simulink subsystem "RT_HubLinearAndAngularVelocity"  (R2025a)
settings: Solver=VariableStepAuto  StartTime=0.0  StopTime=10.0  RelTol=1e-3
settings Model: DataDictionary=Helicopter.sldd  EnableAccessToBaseWorkspace=off  DefaultTestHarness=RT_HubLinearAndAngularVelocity_Harness6  Creator=Admin  LastModifiedBy=Admin

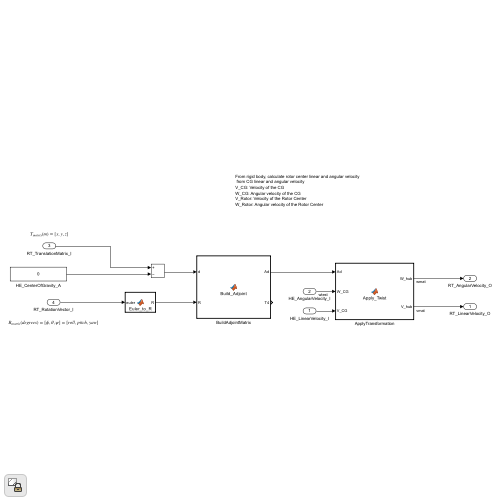
[thumbnail: Simulink's stored preview of the top-level diagram]
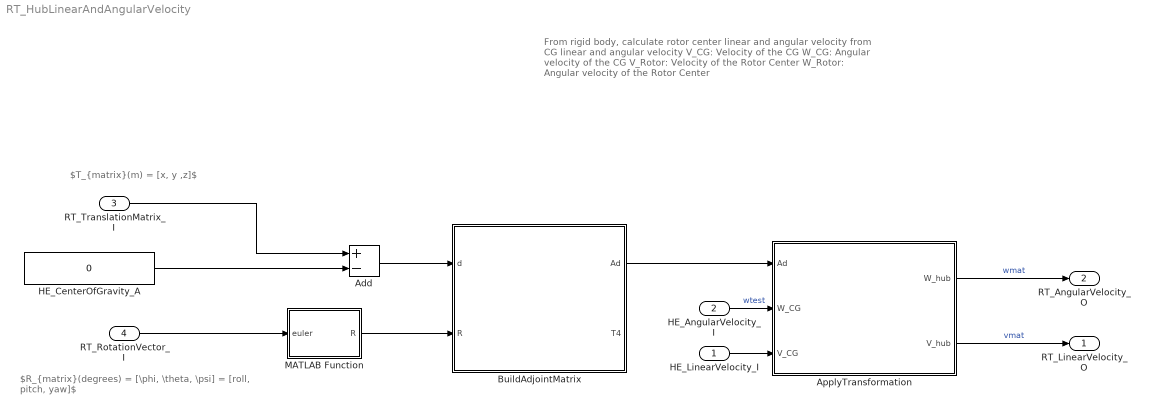
== system RT_HubLinearAndAngularVelocity ==
  note: From rigid body, calculate rotor center linear and angular velocity
      |  from CG linear and angular velocity
      | V_CG: Velocity of the CG
      | W_CG: Angular velocity of the CG
      | V_Rotor: Velocity of the Rotor Center
      | W_Rotor: Angular velocity of the Rotor Center
  note: $R_{matrix}(degrees) = [\phi, \theta, \psi] = [roll, pitch, yaw]$
  note: $T_{matrix}(m) = [x, y ,z]$
  HE_LinearVelocity_I : Inport
  HE_AngularVelocity_I : Inport  Port=2
  RT_TranslationMatrix_I : Inport  Port=3
  RT_RotationVector_I : Inport  Port=4
  Add : Sum  Inputs=+-
  ApplyTransformation : MATLAB Function  TreatAsAtomicUnit=on
  BuildAdjointMatrix : MATLAB Function  TreatAsAtomicUnit=on
  HE_CenterOfGravity_A : Constant  Value=0
  MATLAB Function : MATLAB Function  TreatAsAtomicUnit=on
  RT_LinearVelocity_O : Outport
  RT_AngularVelocity_O : Outport  Port=2
  wires:
  HE_CenterOfGravity_A/1 -> Add/2
  ApplyTransformation/1(W_hub) -> RT_AngularVelocity_O/1  "wmat"
  RT_TranslationMatrix_I/1 -> Add/1
  ApplyTransformation/2(V_hub) -> RT_LinearVelocity_O/1  "vmat"
  Add/1 -> BuildAdjointMatrix/1(d)
  HE_LinearVelocity_I/1 -> ApplyTransformation/3(V_CG)
  MATLAB Function/1(R) -> BuildAdjointMatrix/2(R)
  HE_AngularVelocity_I/1 -> ApplyTransformation/2(W_CG)  "wtest"
  RT_RotationVector_I/1 -> MATLAB Function/1(euler)
  BuildAdjointMatrix/1(Ad) -> ApplyTransformation/1(Ad)

== matlab function RT_HubLinearAndAngularVelocity/ApplyTransformation ==
  data: Ad input; W_CG input; W_hub output; V_CG input; V_hub output
function [W_hub, V_hub] = Apply_Twist(Ad,W_CG, V_CG)
%APPLY_TWIST  Applies the 6x6 Adjoint to transform a velocity twist
%             from CG frame to hub frame.
%
%   Input  twist at CG:  [W_CG (3x1); V_CG (3x1)]
%   Output twist at hub: [W_hub(3x1); V_hub(3x1)]

twist_CG  = [W_CG; V_CG];       % stack into 6x1
twist_hub = Ad * twist_CG;       % single matrix multiply

W_hub = twist_hub(1:3);
V_hub = twist_hub(4:6);

== matlab function RT_HubLinearAndAngularVelocity/BuildAdjointMatrix ==
  data: d input; Ad output; R input; T4 output
function [Ad, T4] = Build_Adjoint(d, R)
%BUILD_ADJOINT  Forms velocity Adjoint, wrench Adjoint, and homogeneous transform.
%
%   Velocity transform  (twist):   [W_hub; V_hub]   = Ad        * [W_CG;  V_CG]

% ── Skew-symmetric matrix ─────────────────────────────────────────────
S = [  0     -d(3)   d(2);
       d(3)   0     -d(1);
      -d(2)   d(1)   0   ];

% ── Velocity Adjoint (as before) ──────────────────────────────────────
%   [W_hub; V_hub] = Ad * [W_CG; V_CG]
Ad = [ R,        zeros(3);
      -R*S,      R          ];

% ── Homogeneous transform (geometry only) ─────────────────────────────
T4 = [ R,  d;
       0, 0, 0, 1 ];

== matlab function RT_HubLinearAndAngularVelocity/MATLAB Function ==
  data: euler input; R output
function R = Euler_to_R(euler)

phi   = euler(1);
theta = euler(2);
psi   = euler(3);

% Precompute trig
cp = cos(phi);   sp = sin(phi);
ct = cos(theta); st = sin(theta);
cy = cos(psi);   sy = sin(psi);

% ZYX expanded form — standard aerospace rotation matrix
R = [ cy*ct,   cy*st*sp - sy*cp,   cy*st*cp + sy*sp;
      sy*ct,   sy*st*sp + cy*cp,   sy*st*cp - cy*sp;
     -st,      ct*sp,              ct*cp            ]';
